simulink model "Day2_2_average_filter"  (R2022b)
settings: Solver=FixedStepAuto  StartTime=0.0  StopTime=10.0  FixedStep=0.001  RelTol=1e-3
settings Model: Creator=user  LastModifiedBy=user

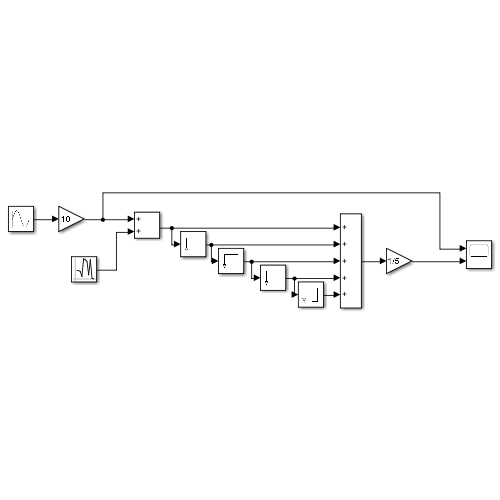
[thumbnail: Simulink's stored preview of the top-level diagram]
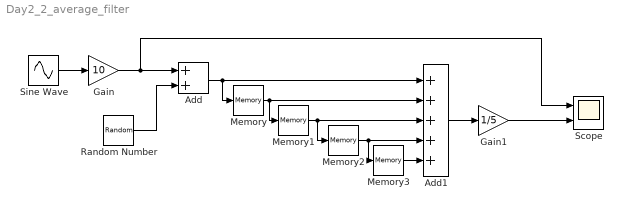
== system Day2_2_average_filter ==
  Add : Sum
  Add1 : Sum  Inputs=+++++
  Gain : Gain  Gain=10
  Gain1 : Gain  Gain=1/5
  Memory{,1..3} (4 alike) : Memory
  Random Number : RandomNumber  SampleTime=0.001
  Scope : Scope  NumInputPorts=2
  Sine Wave : Sin  Frequency=0.25*2*pi  SampleTime=0
  wires:
  Sine Wave/1 -> Gain/1
  Gain/1 -> Scope/1, Add/1
  Random Number/1 -> Add/2
  Add/1 -> Memory/1, Add1/1
  Memory/1 -> Memory1/1, Add1/2
  Memory1/1 -> Memory2/1, Add1/3
  Memory2/1 -> Memory3/1, Add1/4
  Memory3/1 -> Add1/5
  Add1/1 -> Gain1/1
  Gain1/1 -> Scope/2
